simulink model "interdistance_control"  (R2021a)
settings: Solver=VariableStepAuto  StartTime=0.0  StopTime=10.0  RelTol=1e-3  EnableMultiTasking=on
libraries: pid_lib x1, fuzblock x1, Driver_Glider_Library x1
settings Model: Creator=HP  LastModifiedBy=HP
settings SolverCC: AlgebraicLoopSolver=TrustRegion
settings DataIOCC: ReturnWorkspaceOutputs=off
settings OptimizationCC: LifeSpan=inf
settings DebuggingCC: SFUnexpectedBacktrackingDiag=warning  SFNoUnconditionalDefaultTransitionDiag=warning  SFMachineParentedDataDiag=warning  ArithmeticOperatorsInVariantConditions=warning
settings SFSimCC: SimUseLocalCustomCode=off  CustomCodeUndefinedFunction=UseInterfaceOnly
settings RTWCC: RTWUseLocalCustomCode=off
settings CodeAppCC: StateflowObjectComments=on
settings GRTTargetCC: TargetLangStandard=C89/C90 (ANSI)
settings ConfigComp: CovMetricSettings=dw  CovSaveCumulativeToWorkspaceVar=on  CovSaveSingleToWorkspaceVar=on  CovExternalEMLEnable=off

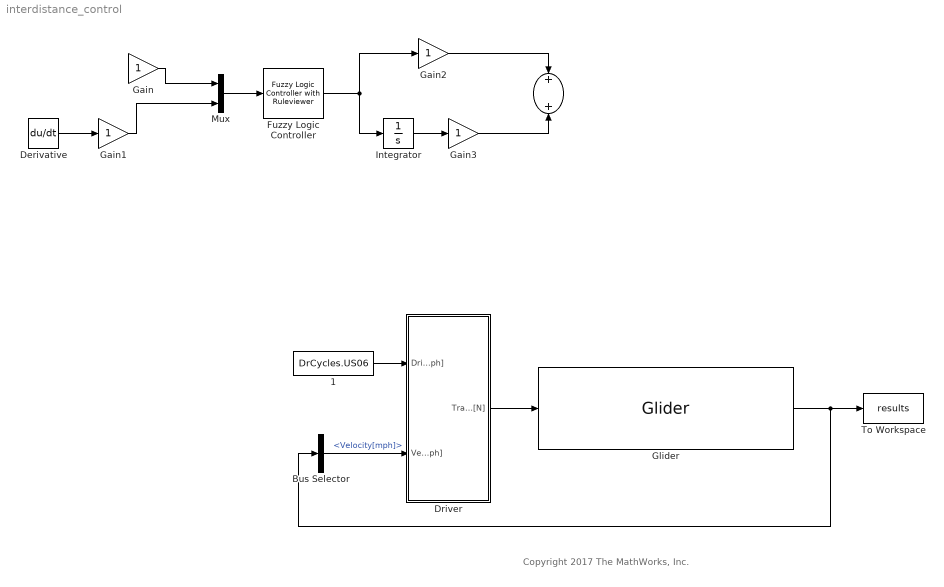
== system interdistance_control ==
  note: Copyright 2017 The MathWorks, Inc.
  " 1" : FromWorkspace  Tag=DriveCycle  VariableName=DrCycles.US06
  " " : Sum
  Bus Selector : BusSelector  OutputSignals=Velocity[mph]
  Derivative : Derivative
  Driver : Subsystem
      mask Display: image('DriverPic.jpg');
  "Fuzzy Logic Controller " : fuzblock/Fuzzy Logic  Controller  with Ruleviewer  fismatrix=[]  Ts=2
  Gain{,1..3} (4 alike) : Gain
  Glider : Driver_Glider_Library/Glider  SystemSampleTime=-1  VariantActivationTime=update diagram  Latency=0  AutoFrameSizeCalculation=off
  Integrator : Integrator
  Mux : Mux  Inputs=2
  To Workspace : ToWorkspace  VariableName=results  SaveFormat=Timeseries  SampleTime=-1
  wires:
  Gain/1 -> Mux/1
  Gain1/1 -> Mux/2
  Mux/1 -> "Fuzzy Logic Controller "/1
  Derivative/1 -> Gain1/1
  Gain2/1 -> " "/1
  Gain3/1 -> " "/2
  Integrator/1 -> Gain3/1
  "Fuzzy Logic Controller "/1 -> Integrator/1, Gain2/1
  " 1"/1 -> Driver/1(DriveCycleSpeed[mph])
  Driver/1(TractiveForce[N]) -> Glider/1
  Bus Selector/1 -> Driver/2(VehicleSpeed[mph])  "<Velocity[mph]>"
  Glider/1 -> To Workspace/1, Bus Selector/1

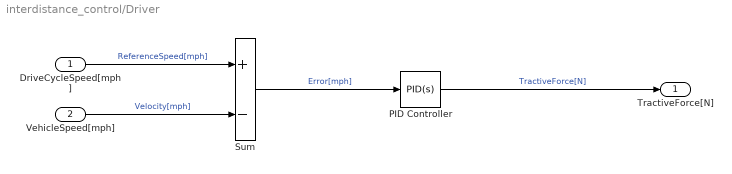
== system interdistance_control/Driver ==
  DriveCycleSpeed[mph] : Inport
  VehicleSpeed[mph] : Inport  Port=2
  PID Controller : pid_lib/PID Controller  Controller=PID  Form=Parallel  TimeDomain=Continuous-time  UseExternalTs=off  SampleTime=-1  IntegratorMethod=Forward Euler  FilterMethod=Forward Euler  ControllerParametersSource=internal  P=7500  I=1  D=0  UseFilter=on  N=100  TunerSelectOption=Transfer Function Based (PID Tuner App)  InitialConditionSource=internal  InitialConditionForIntegrator=0  InitialConditionForFilter=0  DifferentiatorICPrevScaledInput=0  ExternalReset=none  TrackingMode=off  Kt=1  LimitOutput=off  SatLimitsSource=internal  UpperSaturationLimit=inf  LowerSaturationLimit=-inf  LinearizeAsGain=on  AntiWindupMode=none  Kb=1  POutMin=[]  POutMax=[]  IOutMin=[]  IOutMax=[]  DOutMin=[]  DOutMax=[]  NOutMin=[]  NOutMax=[]  SumOutMin=[]  SumOutMax=[]  SaturationOutMin=[]  SaturationOutMax=[]  PParamMin=[]  PParamMax=[]  IParamMin=[]  IParamMax=[]  DParamMin=[]  DParamMax=[]  NParamMin=[]  NParamMax=[]  KbParamMin=[]  KbParamMax=[]  KtParamMin=[]  KtParamMax=[]  KbOutMin=[]  KbOutMax=[]  KtOutMin=[]  KtOutMax=[]  IntegratorOutMin=[]  IntegratorOutMax=[]  FilterOutMin=[]  FilterOutMax=[]  SumI1OutMin=[]  SumI1OutMax=[]  SumI2OutMin=[]  SumI2OutMax=[]  SumI3OutMin=[]  SumI3OutMax=[]  SumI4OutMin=[]  SumI4OutMax=[]  SumDOutMin=[]  SumDOutMax=[]  DifferentiatorOutMin=[]  DifferentiatorOutMax=[]  FilterDiffOutCoefMin=[]  FilterDiffOutCoefMax=[]  ReciprocalOutMin=[]  ReciprocalOutMax=[]  SumDenOutMin=[]  SumDenOutMax=[]  SumNumOutMin=[]  SumNumOutMax=[]  DivideOutMin=[]  DivideOutMax=[]  UdiffTsProdOutMin=[]  UdiffTsProdOutMax=[]  NTsProdOutMin=[]  NTsProdOutMax=[]  UintegralTsProdOutMin=[]  UintegralTsProdOutMax=[]  UngainTsProdOutMin=[]  UngainTsProdOutMax=[]  IntegratorContinuousStateAttributes=''  IntegratorStateMustResolveToSignalObject=off  IntegratorRTWStateStorageClass=Auto  FilterContinuousStateAttributes=''  FilterStateMustResolveToSignalObject=off  FilterRTWStateStorageClass=Auto  ParallelPVariant=InternalParameters  IdealPVariant=Disabled  IVariant=InternalParameters  DVariant=InternalParameters  IntegratorVariant=Continuous  SatVariant=Disabled  AWVariant=Passthrough  PCopyVariant=Disabled  TRVariant=Disabled  FdbkBlocksVariant=Forward  IdealPFdbkVariant=Disabled  SatFdbkVariant=Disabled  DerivativeFilterVariant=ContFilter  NVariant=InternalParameters  NCopyVariant=Disabled  FilterICVariant=InternalICsFilter  IntegratorICVariant=InternalICs  ExternalResetVariant=Disabled  TRSumVariant=Passthrough  SumFdbkVariant=Disabled  SumVariant=Sum_PID  TsampFilterVariant=InternalTs  TsampNgainVariant=Passthrough  TsampIntegralVariant=Passthrough  ExternalSaturationOutDataTypeStr=Inherit: Same as second input
  Sum : Sum  Inputs=+-
  TractiveForce[N] : Outport  VectorParamsAs1DForOutWhenUnconnected=off
  wires:
  DriveCycleSpeed[mph]/1 -> Sum/1  "ReferenceSpeed[mph]"
  Sum/1 -> PID Controller/1  "Error[mph]"
  VehicleSpeed[mph]/1 -> Sum/2  "Velocity[mph]"
  PID Controller/1 -> TractiveForce[N]/1  "TractiveForce[N]"
